simulink model "ratio_esc_closed_loop"  (R2022b)
settings: Solver=FixedStepDiscrete  StartTime=0.0  StopTime=599.95000000000005  FixedStep=0.050000000000000003  RelTol=1e-3
model workspace (MAT data in the model file):
  noise_input = [0 0.05 0.1 0.15 0.2 0.25 0.3 0.35 0.4 0.45 0.5 0.55 ... (24000 elements, 12000x2)]
  optimum_input = [0 0.05 0.1 0.15 0.2 0.25 0.3 0.35 0.4 0.45 0.5 0.55 ... (24000 elements, 12000x2)]
  ratio_configuration.Ts = 0.05
  ratio_configuration.duration = 600
  ratio_configuration.initialRatio = 1.2
  ratio_configuration.lower = 0.75
  ratio_configuration.upper = 1.25
  ratio_configuration.tau = 0.25
  ratio_configuration.rateLimit = 0.05
  ratio_configuration.amplitude = 0.02
  ratio_configuration.frequency = 0.1
  ratio_configuration.hpOmega = 0.05
  ratio_configuration.lpOmega = 0.05
  ratio_configuration.gain = 0.003
  ratio_configuration.noiseSigma = 0
  ratio_configuration.delay = 0
  ratio_configuration.seed = 1
  ratio_configuration.stage = 'esc'
  ratio_configuration.scenario = 'stationary'
  ratio_configuration.fixedReference = 0.95
  ratio_configuration.optimalRatio = 0.9
  ratio_configuration.shiftedOptimalRatio = 1.05
  ratio_configuration.shiftTime = 300
  ratio_configuration.curvature = 4
  ratio_configuration.rlPeriod = 1
libraries: simulink x1
(part 1 of 2)
settings Model: Creator=偷走月亮的猫  LastModifiedBy=偷走月亮的猫

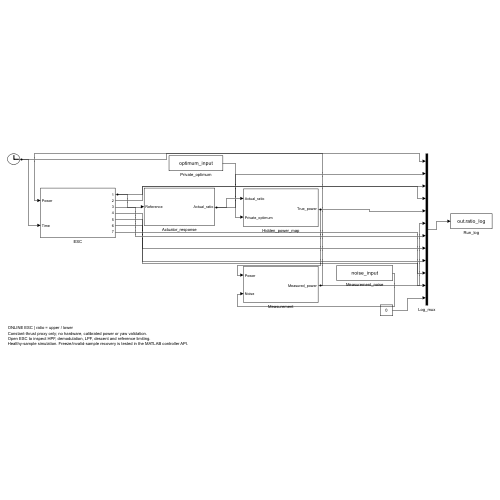
[thumbnail: Simulink's stored preview of the top-level diagram]
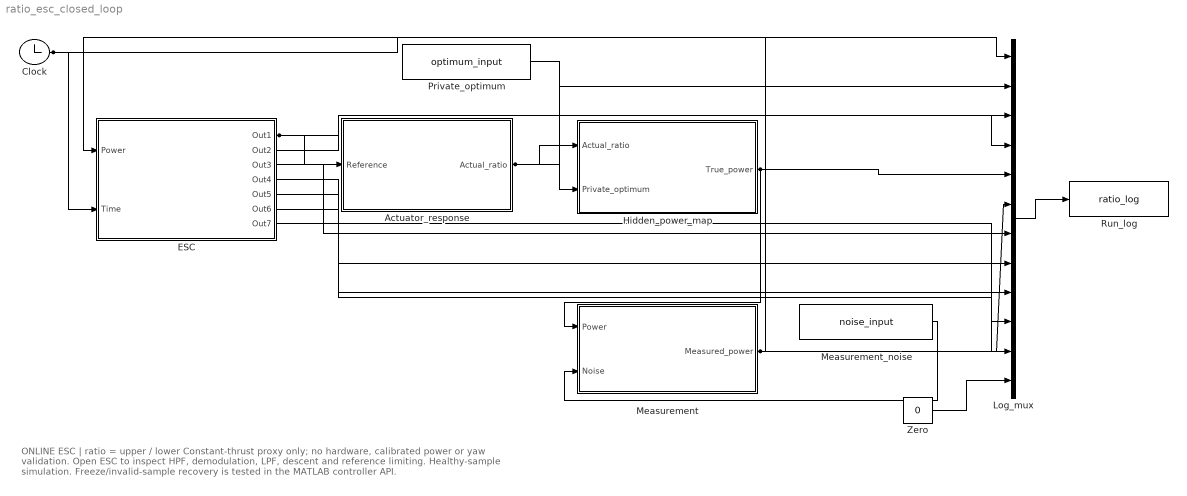
== system ratio_esc_closed_loop ==
  note: ONLINE ESC | ratio = upper / lower
      | Constant-thrust proxy only; no hardware, calibrated power or yaw validation.
      | Open ESC to inspect HPF, demodulation, LPF, descent and reference limiting.
      | Healthy-sample simulation. Freeze/invalid-sample recovery is tested in the MATLAB controller API.
  Actuator_response : Subsystem
  Clock : Clock
  ESC : Subsystem
  Hidden_power_map : Subsystem
  Log_mux : Mux  Inputs=12
  Measurement : Subsystem
  Measurement_noise : FromWorkspace  VariableName=noise_input  Interpolate=off  OutputAfterFinalValue=Holding final value
  Private_optimum : FromWorkspace  VariableName=optimum_input  Interpolate=off  OutputAfterFinalValue=Holding final value
  Run_log : ToWorkspace  VariableName=ratio_log  SampleTime=-1
  Zero : Constant  Value=0
  wires:
  Clock/1 -> ESC/2(Time), Log_mux/1
  ESC/1(Out1) -> Actuator_response/1(Reference), Log_mux/3
  Actuator_response/1(Actual_ratio) -> Hidden_power_map/1(Actual_ratio), Log_mux/2
  Private_optimum/1 -> Hidden_power_map/2(Private_optimum)
  Hidden_power_map/1(True_power) -> Measurement/1(Power), Log_mux/5
  Measurement_noise/1 -> Measurement/2(Noise)
  Measurement/1(Measured_power) -> ESC/1(Power), Log_mux/6
  ESC/2(Out2) -> Log_mux/4
  ESC/3(Out3) -> Log_mux/7
  ESC/4(Out4) -> Log_mux/8
  ESC/5(Out5) -> Log_mux/9
  ESC/6(Out6) -> Log_mux/10
  ESC/7(Out7) -> Log_mux/11
  Zero/1 -> Log_mux/12
  Log_mux/1 -> Run_log/1
